simulink library "AK_snowman_library"  (R2023b)
settings: Solver=VariableStepAuto  StartTime=0.0  StopTime=10.0  RelTol=1e-3
settings Model: LastModifiedBy=mluser

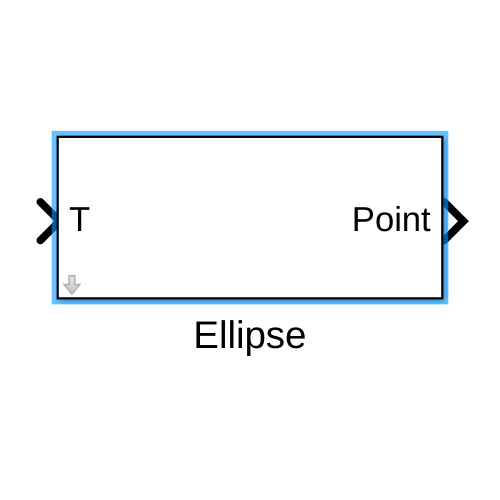
[thumbnail: Simulink's stored preview of the top-level diagram]
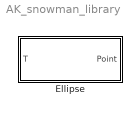
== system AK_snowman_library ==
  Ellipse : Subsystem  mask{X_offset=0, Y_offset=0, A=0, B=0}
      mask prompts: X_offset "X offset"; Y_offset "Y offset"
      mask DialogControl DescTextVar Prompt: %<MaskDescription> A is the radius of x, B is the radius of y

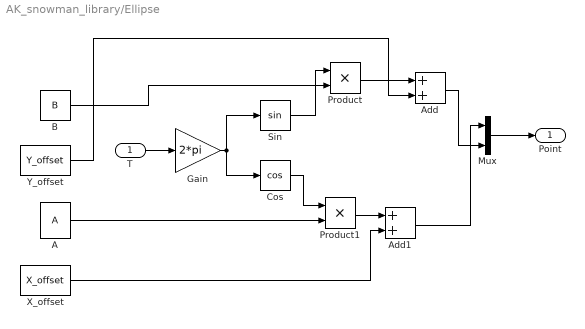
== system AK_snowman_library/Ellipse ==
  T : Inport
  A : Constant  Value=A
  Add : Sum
  Add1 : Sum
  B : Constant  Value=B
  Cos : Trigonometry  Operator=cos
  Gain : Gain  Gain=2*pi
  Mux : Mux  Inputs=2
  Product : Product
  Product1 : Product
  Sin : Trigonometry
  X_offset : Constant  Value=X_offset
  Y_offset : Constant  Value=Y_offset
  Point : Outport
  wires:
  Y_offset/1 -> Add/2
  Product/1 -> Add/1
  X_offset/1 -> Add1/2
  Add1/1 -> Mux/1
  Cos/1 -> Product1/1
  B/1 -> Product/2
  A/1 -> Product1/2
  Sin/1 -> Product/1
  Gain/1 -> Cos/1, Sin/1
  Product1/1 -> Add1/1
  T/1 -> Gain/1
  Add/1 -> Mux/2
  Mux/1 -> Point/1
